simulink model "test_co"  (R2019a)
settings: Solver=VariableStepAuto  StartTime=0.0  StopTime=10.0  RelTol=1e-3
settings Model: Creator=ardui  LastModifiedBy=ardui

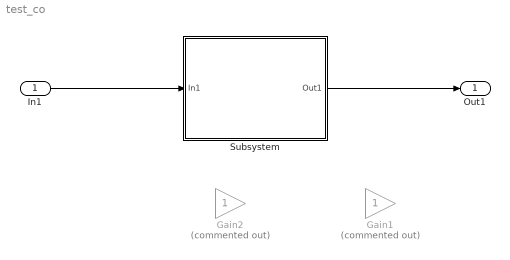
== system test_co ==
  In1 : Inport
  Gain1 : Gain  Commented=on
  Gain2 : Gain  Commented=on
  Subsystem : Subsystem
  Out1 : Outport
  wires:
  In1/1 -> Subsystem/1(In1)
  Subsystem/1(Out1) -> Out1/1

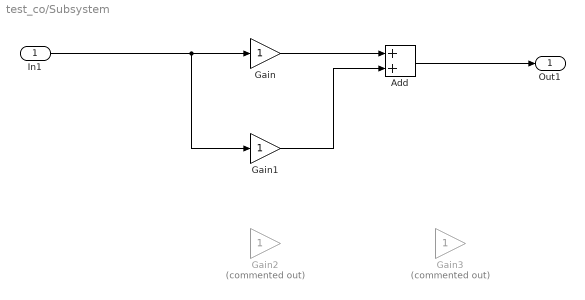
== system test_co/Subsystem ==
  In1 : Inport
  Add : Sum
  Gain : Gain
  Gain1 : Gain
  Gain2 : Gain  Commented=on
  Gain3 : Gain  Commented=on
  Out1 : Outport
  wires:
  Gain/1 -> Add/1
  In1/1 -> Gain1/1, Gain/1
  Gain1/1 -> Add/2
  Add/1 -> Out1/1
